simulink model "StagingTest"  (R2015a)
settings: Solver=ode45  StartTime=0.0  StopTime=20  RelTol=1e-3
libraries: dspswit3 x1
settings Model: Creator=raulm_000  LastModifiedBy=raulm_000

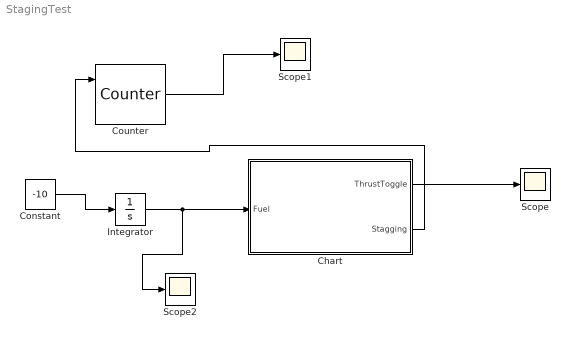
== system StagingTest ==
  Chart : Stateflow chart  TreatAsAtomicUnit=on
  Constant : Constant  Value=-10
  Counter : dspswit3/Counter  Direction=Up  CountEvent=Rising edge  CounterSize=User defined  MaxCount=5  InitialCount=1  Output=Count  HitValue=5  ResetInput=on  SamplesPerFrame=1  Ts=1  CntDtype=double  HitDtype=Logical
  Integrator : Integrator  InitialCondition=100  LimitOutput=on  LowerSaturationLimit=0
  Scope : Scope
  Scope1 : Scope
  Scope2 : Scope
      settings: SaveName=ScopeData2
  wires:
  Integrator/1 -> Scope2/1, Chart/1(Fuel)
  Constant/1 -> Integrator/1
  Chart/2(Stagging) -> Counter/1
  Chart/1(ThrustToggle) -> Scope/1
  Counter/1 -> Scope1/1

== stateflow chart StagingTest/Chart ==
  settings: initializeOutput=1
  state Nominal
    entry: ThrustToggle = 1
    entry: Stagging = 0
  state Stage_Rocket
    entry: ThrustToggle = 0
    entry: Stagging = 1
  (default) -> Nominal
  Nominal -> Stage_Rocket : {Fuel == 0}
  Stage_Rocket -> Nominal : [Fuel > 0]
  data: Fuel input; ThrustToggle output; Stagging output
